simulink model "PushPull"  (R2012b)
settings: Solver=ode1  StartTime=0.0  StopTime=12  FixedStep=.001  RelTol=1e-3
undefined symbols (not defined in the file): HIL, LCconv
libraries: quarc_library x5, simulink x1
settings Model: SimulationMode=external  ExtModeTrigDuration=5000000  Creator=LabUser  LastModifiedBy=LabUser
settings SolverCC: PositivePriorityOrder=on
settings DataIOCC: LimitDataPoints=off
settings DebuggingCC: SolverPrmCheckMsg=none
settings RTWCC: SystemTargetFile=quarc_win64.tlc  TemplateMakefile=quarc_default_tmf  Description=QUARC Win64 Target  ProcessScript=quarc_win64_make_rtw_hook
settings STFCustomTargetCC: TargetPreCompLibLocation=C:\PROGRA~3\QUARC\lib\2012b\win64\release  CodeReplacementLibrary=ANSI_C  GeneratePreprocessorConditionals=Disable all  CombineOutputUpdateFcns=on  GRTInterface=off  SystemTargetFile=quarc_win64.tlc
settings GRTTargetCC: TargetPreCompLibLocation=C:\PROGRA~3\QUARC\lib\2012b\win64\release  ParMdlRefBuildCompliant=off  CompOptLevelCompliant=off  ConcurrentExecutionCompliant=off  MatFileLogging=off  ExtMode=on  ExtModeMexFile=quarc_comm

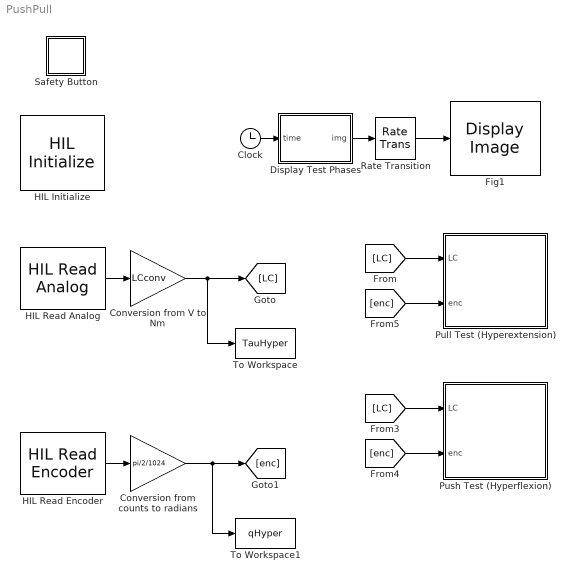
== system PushPull ==
  Clock : Clock
  Conversion from V to Nm : Gain  Gain=LCconv
  Conversion from counts to radians : Gain  Gain=pi/2/1024
  Display Test Phases : MATLAB Function  TreatAsAtomicUnit=on
  "Fig1 " : quarc_library/Sinks/Figures/Display Image  figure_mode=Use figure window  figure_tag=figure1  axes_tag=axes1  update_rate=1  initial_position="9  580  624  385"  initial_visibility=on  sample_time=0.1
  HIL Initialize : quarc_library/Data Acquisition/Generic/Configuration/HIL Initialize  Priority=-99  object_name=HIL-1  board_type=qpid_e  board_number=0  board_options=enc0_dir=0;enc0_filter=1;enc0_a=1;enc0_b=1;enc0_z=0;enc0_reload=0;enc1_dir=0;enc1_filter=1;enc1_a=1;enc1_b=1;enc1_z=0;enc1_reload=0;enc2_dir=0;enc2_filter=1;enc2_a=1;enc2_b=1;enc2_z=0;enc2_reload=0;enc3_dir=0;enc3_filter=1;enc3_a=1;enc3_b=1;enc3_z=0;enc3_reload=0;enc4_dir=0;enc4_filter=1;enc4_a=1;enc4_b=1;enc4_z=0;enc4_reload=0;enc5_dir=0;enc5_filter=1;enc5_a=1;enc5_b=1;enc5_z=0;enc5_reload=0;enc6_dir=0;enc6_filter=1;enc6_a=1;enc6_b=1;enc6_z=0;enc6_reload=0;enc7_dir=0;enc7_filter=1;enc7_a=1;enc7_b=1;enc7_z=0;enc7_reload=0;ext_int_polarity=0;fuse_polarity=0;convert_polarity=0;watchdog_polarity=0;ext_int_watchdog=0;fuse_watchdog=0;trig1_watchdog=0;watchdog_to_trig1=0;watchdog_to_trig2=0;counter_to_trig0=0;trigger_adcs=0;latch_on_adc=0;pwm_immediate=0  exclusive=off  active=off  hardware_clocks=[0:16]  clock_modes=[]  initial_clock_frequencies=[]  set_clock_params_at_start=off  set_clock_params_at_switch_in=off  set_clock_frequencies_at_start=off  set_clock_frequencies_at_switch_in=off  analog_input_channels=[0:7]  analog_input_maximums=10  analog_input_minimums=-10  set_analog_input_params_at_start=off  set_analog_input_params_at_switch_in=off  analog_output_channels=[0:7]  analog_output_maximums=10  analog_output_minimums=-10  initial_analog_outputs=[0]  final_analog_outputs=[0]  watchdog_analog_outputs=0  set_analog_output_params_at_start=off  set_analog_output_params_at_switch_in=off  set_analog_outputs_at_start=on  set_analog_outputs_at_switch_in=off  set_analog_outputs_at_terminate=on  set_analog_outputs_at_switch_out=off  set_analog_outputs_on_watchdog=off  digital_input_channels=[]  digital_output_channels=[]  digital_output_configuration=[]  initial_digital_outputs=[1]  final_digital_outputs=[1]  watchdog_digital_outputs=[2]  set_digital_output_params_at_start=off  set_digital_output_params_at_switch_in=off  set_digital_outputs_at_start=on  set_digital_outputs_at_switch_in=off  set_digital_outputs_at_terminate=on  set_digital_outputs_at_switch_out=off  set_digital_outputs_on_watchdog=off  encoder_channels=[0:7]  quadrature=[4]  encoder_filter_frequency=40e6/1  initial_encoder_counts=[0]  set_encoder_params_at_start=on  set_encoder_params_at_switch_in=off  set_encoder_counts_at_start=off  set_encoder_counts_at_switch_in=off  pwm_channels=[0:7]  pwm_modes=0  pwm_frequency=40e6/4096  pwm_configuration=[0]  pwm_alignment=[0]  pwm_polarity=[1]  pwm_leading_deadband=[0]  pwm_trailing_deadband=[0]  initial_pwm_outputs=[0]  final_pwm_outputs=[0]  watchdog_pwm_outputs=[0]  set_pwm_params_at_start=on  set_pwm_params_at_switch_in=off  set_pwm_outputs_at_start=on  set_pwm_outputs_at_switch_in=off  set_pwm_outputs_at_terminate=on  set_pwm_outputs_at_switch_out=off  set_pwm_outputs_on_watchdog=off  other_output_channels=[]  initial_other_outputs=[]  final_other_outputs=[]  watchdog_other_outputs=[]  set_other_outputs_at_start=off  set_other_outputs_at_switch_in=off  set_other_outputs_at_terminate=off  set_other_outputs_at_switch_out=off  set_other_outputs_on_watchdog=off
  HIL Read Analog : quarc_library/Data Acquisition/Generic/Immediate I//O/HIL Read Analog  object_name=HIL-1  channels=0  sample_time=qc_get_step_size  active=on  vector_output=off
  HIL Read Encoder : quarc_library/Data Acquisition/Generic/Immediate I//O/HIL Read Encoder  object_name=HIL-1  channels=0  sample_time=qc_get_step_size  active=on  vector_output=off  data_type_mode=Inherit via back propagation  data_type=double
  Pull Test (Hyperextension) : Subsystem
  Push Test (Hyperflexion) : Subsystem
  Rate Transition : RateTransition  X0=reshape([zeros(100,100,1),zeros(100,100,1),256*ones(100,100,1)],100,100,3)  OutPortSampleTime=.1
  Safety Button : Subsystem
  To Workspace : ToWorkspace  VariableName=TauHyper  SampleTime=-1
  To Workspace1 : ToWorkspace  VariableName=qHyper  SampleTime=-1
  wires:
  HIL Read Analog/1 -> Conversion from V to Nm/1
  Conversion from V to Nm/1 -> To Workspace/1, [LC]
  HIL Read Encoder/1 -> Conversion from counts to radians/1
  Conversion from counts to radians/1 -> To Workspace1/1, [enc]
  [enc] -> Pull Test (Hyperextension)/2(enc)
  [LC] -> Pull Test (Hyperextension)/1(LC)
  [enc] -> Push Test (Hyperflexion)/2(enc)
  [LC] -> Push Test (Hyperflexion)/1(LC)
  Clock/1 -> Display Test Phases/1(time)
  Display Test Phases/1(img) -> Rate Transition/1
  Rate Transition/1 -> "Fig1 "/1

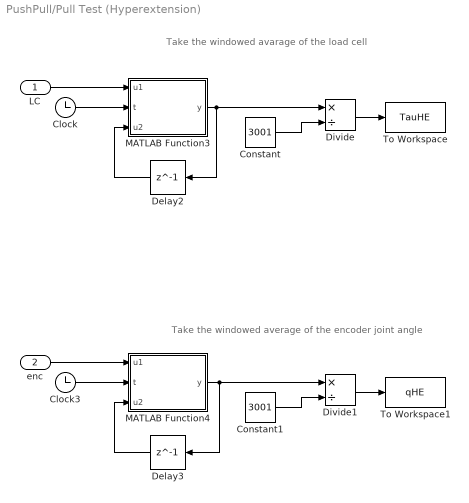
== system PushPull/Pull Test (Hyperextension) ==
  note: Take the windowed avarage of the load cell
  note: Take the windowed average of the encoder joint angle
  LC : Inport
  enc : Inport  Port=2
  Clock : Clock
  Clock3 : Clock
  Constant : Constant  Value=3001
  Constant1 : Constant  Value=3001
  Delay2 : Delay  DelayLength=1  InitialCondition=0
  Delay3 : Delay  DelayLength=1  InitialCondition=0
  Divide : Product  Inputs=*/
  Divide1 : Product  Inputs=*/
  MATLAB Function3 : MATLAB Function  TreatAsAtomicUnit=on
  MATLAB Function4 : MATLAB Function  TreatAsAtomicUnit=on
  To Workspace : ToWorkspace  VariableName=TauHE  SampleTime=-1
      settings: MaxDataPoints=1
  To Workspace1 : ToWorkspace  VariableName=qHE  SampleTime=-1
      settings: MaxDataPoints=1
  wires:
  MATLAB Function3/1(y) -> Divide/1, Delay2/1
  Constant/1 -> Divide/2
  MATLAB Function4/1(y) -> Delay3/1, Divide1/1
  Constant1/1 -> Divide1/2
  Clock/1 -> MATLAB Function3/2(t)
  LC/1 -> MATLAB Function3/1(u1)
  Delay2/1 -> MATLAB Function3/3(u2)
  Clock3/1 -> MATLAB Function4/2(t)
  enc/1 -> MATLAB Function4/1(u1)
  Delay3/1 -> MATLAB Function4/3(u2)
  Divide/1 -> To Workspace/1
  Divide1/1 -> To Workspace1/1

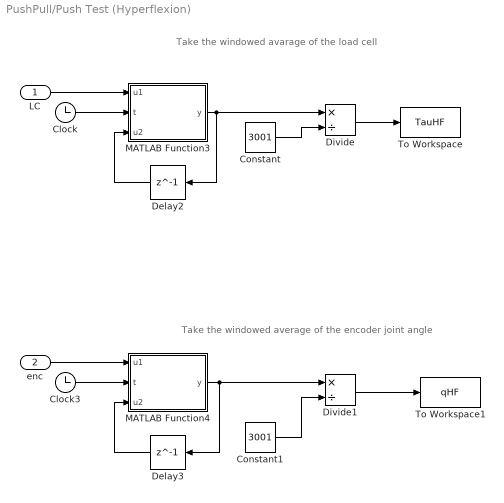
== system PushPull/Push Test (Hyperflexion) ==
  note: Take the windowed avarage of the load cell
  note: Take the windowed average of the encoder joint angle
  LC : Inport
  enc : Inport  Port=2
  Clock : Clock
  Clock3 : Clock
  Constant : Constant  Value=3001
  Constant1 : Constant  Value=3001
  Delay2 : Delay  DelayLength=1  InitialCondition=0
  Delay3 : Delay  DelayLength=1  InitialCondition=0
  Divide : Product  Inputs=*/
  Divide1 : Product  Inputs=*/
  MATLAB Function3 : MATLAB Function  TreatAsAtomicUnit=on
  MATLAB Function4 : MATLAB Function  TreatAsAtomicUnit=on
  To Workspace : ToWorkspace  VariableName=TauHF  SampleTime=-1
      settings: MaxDataPoints=1
  To Workspace1 : ToWorkspace  VariableName=qHF  SampleTime=-1
      settings: MaxDataPoints=1
  wires:
  MATLAB Function3/1(y) -> Divide/1, Delay2/1
  Constant/1 -> Divide/2
  MATLAB Function4/1(y) -> Delay3/1, Divide1/1
  Constant1/1 -> Divide1/2
  Clock/1 -> MATLAB Function3/2(t)
  LC/1 -> MATLAB Function3/1(u1)
  Delay2/1 -> MATLAB Function3/3(u2)
  Clock3/1 -> MATLAB Function4/2(t)
  enc/1 -> MATLAB Function4/1(u1)
  Delay3/1 -> MATLAB Function4/3(u2)
  Divide/1 -> To Workspace/1
  Divide1/1 -> To Workspace1/1

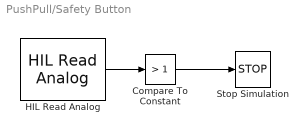
== system PushPull/Safety Button ==
  Compare To Constant : simulink/Logic and Bit Operations/Compare To Constant  relop=>  const=1  OutDataTypeStr=boolean
  HIL Read Analog : quarc_library/Data Acquisition/Generic/Immediate I//O/HIL Read Analog  object_name=HIL-1  channels=[7]  sample_time=qc_get_step_size  active=on  vector_output=off
  Stop Simulation : Stop
  wires:
  HIL Read Analog/1 -> Compare To Constant/1
  Compare To Constant/1 -> Stop Simulation/1

== matlab function PushPull/Display Test Phases ==
  data: time input; img output
function img = fcn(time)

% Image size
w = 100;
if time >= 1 && time < 6 
    % Show image to move to hyperextension.
    r = 0;
    g = 0;
    b = 256;
elseif time >= 6 && time < 11
    % Show image to move to hyperflexion.
    r = 0;
    g = 256;
    b = 0;
elseif time >= 11
    % Release the leg.
    r = 256;
    g = 0;
    b = 0;
else
    % Do nothing (display white)
    r = 256;
    g = 256;
    b = 256;

end

img = reshape([r*ones(w,w,'uint8'),g*ones(w,w,'uint8'),b*ones(w,w,'uint8')],w,w,3);

== matlab function PushPull/Pull Test (Hyperextension)/MATLAB Function3 ==
  data: u1 input; y output; t input; u2 input
function y = fcn(u1,t,u2)

if (t >= 3) && (t <= 6)
    y = u1+u2;
else
    y = u2;
end

== matlab function PushPull/Pull Test (Hyperextension)/MATLAB Function4 ==
  data: u1 input; y output; t input; u2 input
function y = fcn(u1,t,u2)

if (t >= 3) && (t <= 6)
    y = u1+u2;
else
    y = u2;
end

== matlab function PushPull/Push Test (Hyperflexion)/MATLAB Function3 ==
  data: u1 input; y output; t input; u2 input
function y = fcn(u1,t,u2)

if (t >= 8) && (t <= 11)
    y = u1+u2;
else
    y = u2;
end

== matlab function PushPull/Push Test (Hyperflexion)/MATLAB Function4 ==
  data: u1 input; y output; t input; u2 input
function y = fcn(u1,t,u2)

if (t >= 8) && (t <= 11)
    y = u1+u2;
else
    y = u2;
end
